simulink model "sm_backhoe"  (R2021b)
settings: Solver=ode23t  StartTime=0.0  StopTime=60  MaxStep=0.1  RelTol=1e-3  EnableMultiTasking=on
model workspace (MATLAB code in the model file):
  | cylinderGray = [0.6 0.6 0.6];
  | darkOrange = [0.8 0.5 0];
  | glassBlue = [0.2 0.2 1];
  | gray = [0.3 0.3 0.3];
  | orange = [0.8 0.65 0];
  | pistonGray = [0.4 0.4 0.4];
  | tireBlack = [0.1 0.1 0.1];
  | wheelGray = [0.6 0.6 0.6];
  | yellow = [0.8 0.8 0];
  | 
  | rhoGlass = 2500;
  | rhoRubber = 1500;
  | rhoSteel = 7800;
undefined symbols (not defined in the file): sigbuilder_block, X, Y, Z
libraries: sm_lib x161, sm_backhoe_lib x38, nesl_utility x9
(part 1 of 5)
Description:
  | Backhoe
  | 
  | This example shows a hydraulically actuated backhoe model with closed-loop PID control. The mechanism consists of a fixed vehicle model with a base mounting bracket. The bracket allows the backhoe arm to swivel left and right. Additionally, this arm has three rotational degrees of freedom for controlling the position of the bucket relative to the base swivel point.
  | 
  | The backhoe is actuated using pressure inputs to linear acting hydraulic cylinders. Pressure is controlled with decoupled PID controllers that  act on the error between measured and reference angular positions.
settings Model: Creator=The MathWorks, Inc.  LastModifiedBy=The MathWorks, Inc.
settings SolverCC: AlgebraicLoopSolver=TrustRegion  SolverResetMethod=Robust
settings DataIOCC: LimitDataPoints=on  SaveFormat=Array  SaveOutput=off  SaveTime=off  ReturnWorkspaceOutputs=off  Refine=3
settings OptimizationCC: ExpressionDepthLimit=2147483647  LifeSpan=inf
settings DebuggingCC: UnderspecifiedInitializationDetection=Classic  MergeDetectMultiDrivingBlocksExec=none  StateNameClashWarn=warning  SFUnexpectedBacktrackingDiag=warning  SFNoUnconditionalDefaultTransitionDiag=warning  SFExecutionAtInitializationDiag=none  SFMachineParentedDataDiag=warning  ArithmeticOperatorsInVariantConditions=warning
settings HardwareCC: ProdBitPerPointer=32  ProdBitPerSizeT=32  ProdBitPerPtrDiffT=32  ProdLargestAtomicFloat=None  ProdIntDivRoundTo=Undefined  ProdEndianess=Unspecified  ProdWordSize=32  ProdHWDeviceType=32-bit Generic
settings ModelReferenceCC: PropagateSignalLabelsOutOfModel=off
settings SFSimCC: SimUseLocalCustomCode=off  CustomCodeUndefinedFunction=UseInterfaceOnly
settings RTWCC: RTWUseLocalCustomCode=off
settings CodeAppCC: StateflowObjectComments=on
settings GRTTargetCC: TargetLangStandard=C89/C90 (ANSI)
settings ConfigComp: CovMetricSettings=dw  CovSaveCumulativeToWorkspaceVar=on  CovSaveSingleToWorkspaceVar=on  CovExternalEMLEnable=off  CovSFcnEnable=off
settings SimscapeCC: SimscapeNormalizeSystem=off  SimscapeLogType=all  SimscapeLogSimulationStatistics=on  SimscapeLogName=simlog_sm_backhoe  SimscapeLogLimitData=off
settings ConfigurationSet: Description=SimMechanics 2G
settings ExplorerConfigSet: InternalSimMechanicsExplorerSettings="<ExplorerConfiguration><canonicalview>default</canonicalview><TilePanel><TileInfo><Tiles Columns=\"1\" Count=\"1\" Rows=\"1\"><Column Left=\"2\" Weight=\"1\"/><Column Left=\"638\"/><Row Top=\"2\" Weight=\"1\"/><Row Top=\"570\"/><Tile Height=\"1\" Width=\"1\" X=\"0\" Y=\"0\"/></Tiles></TileInfo><SceneInfo><SceneViewer><BGColor><R>0.60000002384185791</R><G>0.60000002384185791</G><B>0.60000002384185791</B></BGColor><Camera><Position><X>17.081954992990738</X><Y>-26.191145003137979</Y><Z>19.643565568520032</Z></Position><Center><X>-1.4975646002791232</X><Y>-7.6116254098681191</Y><Z>1.0640459752315596</Z></Center><Up><X>-0.40824829046386307</X><Y>0.40824829046386307</Y><Z>0.81649658092772615</Z></Up><Left>-11.606539788284151</Left><Right>11.606539788284151</Right><Bottom>-11.304127508235643</Bottom><Top>11.304127508235643</Top></Camera></SceneViewer></SceneInfo></TilePanel></ExplorerConfiguration>"

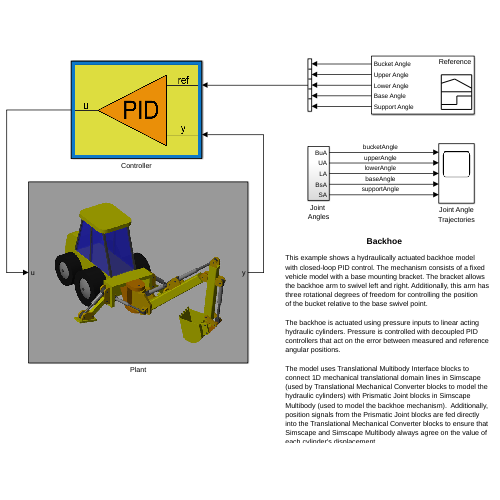
[thumbnail: Simulink's stored preview of the top-level diagram]
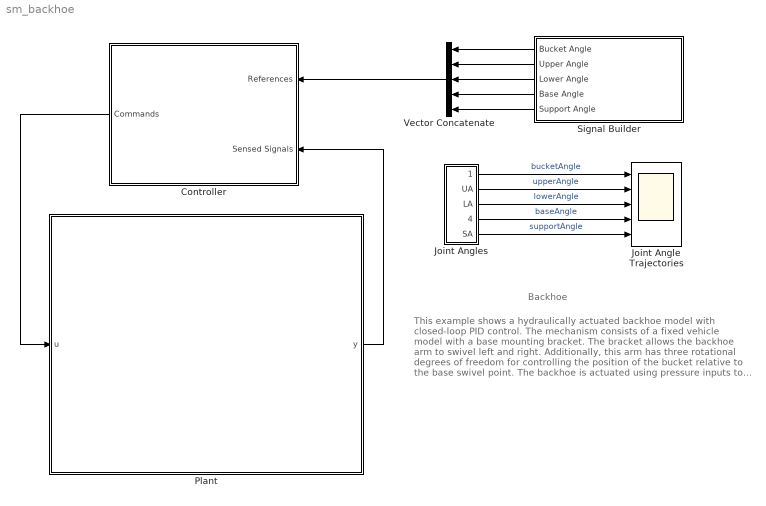
== system sm_backhoe ==
  note: Backhoe
  note: This example shows a hydraulically actuated backhoe model
      | with closed-loop PID control. The mechanism consists of a fixed
      | vehicle model with a base mounting bracket. The bracket allows
      | the backhoe arm to swivel left and right. Additionally, this arm has
      | three rotational degrees of freedom for controlling the position
      | of the bucket relative to the base swivel point.
      |
      | The backhoe is actuated using pressure inputs to linear acting
      | hydraulic cylinders. Pressure is controlled with decoupled PID
      | controllers that act on the error between measured and reference
      | angular positions.
      |
      | The model uses Translational Multibody Interface blocks to
      | connect 1D mechanical translational domain lines in Simscape (used by Translational Mechanical Converter blocks to model the hydraulic cylinders) with Prismatic Joint blocks in Simscape Multibody (used to model the backhoe mechanism).  Additionally, position signals from the Prismatic Joint blocks are fed directly into the Translational Mechanical Converter blocks to ensure that Simscape and Simscape Multibody always agree on the value of each cylinder's displacement.
  Controller : Subsystem
      mask Display: image(fullfile(matlabroot,'toolbox','physmod','sm','smdemos','backhoe','images','sm_backhoe_PIDmask.png'));
  Joint Angles : Subsystem
  Joint Angle Trajectories : Scope  NumInputPorts=5
  Plant : Subsystem
      mask Display:
      | image(fullfile(matlabroot,'toolbox','physmod','sm','smdemos','backhoe','images','sm_backhoe.png'));
      | port_label('input',1,'u');
      | port_label('output',1,'y');
  Signal Builder : Subsystem  Tag=STV Subsys  LoadFcn=sigbuilder_block('load');  StartFcn=sigbuilder_block('start');  StopFcn=sigbuilder_block('stop');  ClipboardFcn=sigbuilder_block('clipboard');  mask(Sigbuilder block){tuvar=[0:10]}
      mask help: Simulink:masks:SigbuilderBlock_MD
      mask init:
      | if ~strcmp(get_param(bdroot(gcbh),'SimulationStatus'),'stopped') tuvar = sigbuilder_block('maskInit'); end
      settings: CopyFcn=sigbuilder_block('copy');  DeleteFcn=sigbuilder_block('delete');  ModelCloseFcn=sigbuilder_block('modelClose');  PreSaveFcn=sigbuilder_block('preSave');  PauseFcn=sigbuilder_block('pause');  ContinueFcn=sigbuilder_block('continue');  NameChangeFcn=sigbuilder_block('namechange');  OpenFcn=sigbuilder_block('open',[252 212.25 471.75 399 ]);  CloseFcn=sigbuilder_block('close');
      mask Display: plot(0, 0, 100, 100,[2, 2, 32, 32, 2], [68, 8, 8, 68, 68],[32, 2], [38, 38], [32, 19, 2],[53, 60, 44], [32, 17, 17, 2],[16, 16, 31, 31]);txt = getActiveGroup(gcbh);text(2, 100, txt,'verticalAlignment', 'top');
  Vector Concatenate : Concatenate  NumInputs=5
  wires:
  Controller/1(Commands) -> Plant/1(u)
  Joint Angles/1(BuA) -> Joint Angle Trajectories/1  "bucketAngle"
  Joint Angles/2(UA) -> Joint Angle Trajectories/2  "upperAngle"
  Joint Angles/3(LA) -> Joint Angle Trajectories/3  "lowerAngle"
  Joint Angles/4(BsA) -> Joint Angle Trajectories/4  "baseAngle"
  Joint Angles/5(SA) -> Joint Angle Trajectories/5  "supportAngle"
  Plant/1(y) -> Controller/2(Sensed Signals)
  Vector Concatenate/1 -> Controller/1(References)
  Signal Builder/2(Upper Angle) -> Vector Concatenate/2
  Signal Builder/3(Lower Angle) -> Vector Concatenate/3
  Signal Builder/1(Bucket Angle) -> Vector Concatenate/1
  Signal Builder/5(Support Angle) -> Vector Concatenate/5
  Signal Builder/4(Base Angle) -> Vector Concatenate/4

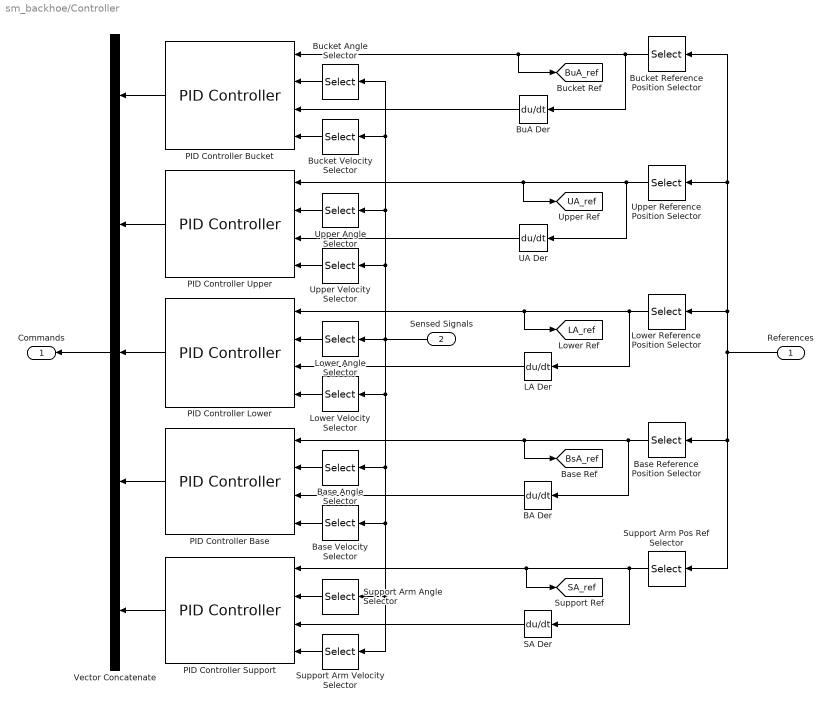
== system sm_backhoe/Controller ==
  References : Inport
  Sensed Signals : Inport  Port=2
  BA Der : Derivative
  Base Angle Selector : Selector  InputPortWidth=10  IndexOptions=Index vector (dialog)  Indices=7  OutputSizes=1
  Base Reference Position Selector : Selector  InputPortWidth=5  IndexOptions=Index vector (dialog)  Indices=4  OutputSizes=1
  Base Velocity Selector : Selector  InputPortWidth=10  IndexOptions=Index vector (dialog)  Indices=8  OutputSizes=1
  BuA Der : Derivative
  Bucket Angle Selector : Selector  InputPortWidth=10  IndexOptions=Index vector (dialog)  Indices=1  OutputSizes=1
  Bucket Reference Position Selector : Selector  InputPortWidth=5  IndexOptions=Index vector (dialog)  Indices=1  OutputSizes=1
  Bucket Velocity Selector : Selector  InputPortWidth=10  IndexOptions=Index vector (dialog)  Indices=2  OutputSizes=1
  LA Der : Derivative
  Lower Angle Selector : Selector  InputPortWidth=10  IndexOptions=Index vector (dialog)  Indices=5  OutputSizes=1
  Lower Reference Position Selector : Selector  InputPortWidth=5  IndexOptions=Index vector (dialog)  Indices=3  OutputSizes=1
  Lower Velocity Selector : Selector  InputPortWidth=10  IndexOptions=Index vector (dialog)  Indices=6  OutputSizes=1
  PID Controller Base : sm_backhoe_lib/PID Controller  upperLim=40  lowerLim=-40  Kp=65  Ki=10  Kd=10
      settings: SourceProductBaseCode=MS
  PID Controller Bucket : sm_backhoe_lib/PID Controller  upperLim=10  lowerLim=-120  Kp=50  Ki=2  Kd=3
      settings: SourceProductBaseCode=MS
  PID Controller Lower : sm_backhoe_lib/PID Controller  upperLim=40  lowerLim=-70  Kp=360  Ki=100  Kd=75
      settings: SourceProductBaseCode=MS
  PID Controller Support : sm_backhoe_lib/PID Controller  upperLim=-40  lowerLim=-100  Kp=40  Ki=1  Kd=2
      settings: SourceProductBaseCode=MS
  PID Controller Upper : sm_backhoe_lib/PID Controller  upperLim=60  lowerLim=-20  Kp=150  Ki=5  Kd=10
      settings: SourceProductBaseCode=MS
  SA Der : Derivative
  Support Arm Angle Selector : Selector  InputPortWidth=10  IndexOptions=Index vector (dialog)  Indices=9  OutputSizes=1
  Support Arm Velocity Selector : Selector  InputPortWidth=10  IndexOptions=Index vector (dialog)  Indices=10  OutputSizes=1
  Support Arm Pos Ref Selector : Selector  InputPortWidth=5  IndexOptions=Index vector (dialog)  Indices=5  OutputSizes=1
  UA Der : Derivative
  Upper Angle Selector : Selector  InputPortWidth=10  IndexOptions=Index vector (dialog)  Indices=3  OutputSizes=1
  Upper Reference Position Selector : Selector  InputPortWidth=5  IndexOptions=Index vector (dialog)  Indices=2  OutputSizes=1
  Upper Velocity Selector : Selector  InputPortWidth=10  IndexOptions=Index vector (dialog)  Indices=4  OutputSizes=1
  Vector Concatenate : Concatenate  NumInputs=5
  Commands : Outport
  tag scope: BsA_ref=global, BuA_ref=global, LA_ref=global, SA_ref=global, UA_ref=global
  wires:
  Vector Concatenate/1 -> Commands/1
  Sensed Signals/1 -> Support Arm Velocity Selector/1, Support Arm Angle Selector/1, Base Velocity Selector/1, Base Angle Selector/1, Lower Velocity Selector/1, Bucket Velocity Selector/1, Bucket Angle Selector/1, Upper Angle Selector/1, Upper Velocity Selector/1, Lower Angle Selector/1
  Upper Angle Selector/1 -> PID Controller Upper/2
  Base Angle Selector/1 -> PID Controller Base/2
  Support Arm Angle Selector/1 -> PID Controller Support/2
  Bucket Angle Selector/1 -> PID Controller Bucket/2
  Lower Angle Selector/1 -> PID Controller Lower/2
  References/1 -> Bucket Reference Position Selector/1, Upper Reference Position Selector/1, Lower Reference Position Selector/1, Support Arm Pos Ref Selector/1, Base Reference Position Selector/1
  PID Controller Support/1 -> Vector Concatenate/5
  Upper Reference Position Selector/1 -> UA Der/1, PID Controller Upper/1, [UA_ref]
  Lower Reference Position Selector/1 -> LA Der/1, [LA_ref], PID Controller Lower/1
  Base Reference Position Selector/1 -> BA Der/1, PID Controller Base/1, [BsA_ref]
  Support Arm Pos Ref Selector/1 -> SA Der/1, [SA_ref], PID Controller Support/1
  Bucket Reference Position Selector/1 -> BuA Der/1, [BuA_ref], PID Controller Bucket/1
  Support Arm Velocity Selector/1 -> PID Controller Support/4
  SA Der/1 -> PID Controller Support/3
  Base Velocity Selector/1 -> PID Controller Base/4
  BA Der/1 -> PID Controller Base/3
  PID Controller Base/1 -> Vector Concatenate/4
  Lower Velocity Selector/1 -> PID Controller Lower/4
  LA Der/1 -> PID Controller Lower/3
  Upper Velocity Selector/1 -> PID Controller Upper/4
  UA Der/1 -> PID Controller Upper/3
  Bucket Velocity Selector/1 -> PID Controller Bucket/4
  BuA Der/1 -> PID Controller Bucket/3
  PID Controller Lower/1 -> Vector Concatenate/3
  PID Controller Upper/1 -> Vector Concatenate/2
  PID Controller Bucket/1 -> Vector Concatenate/1

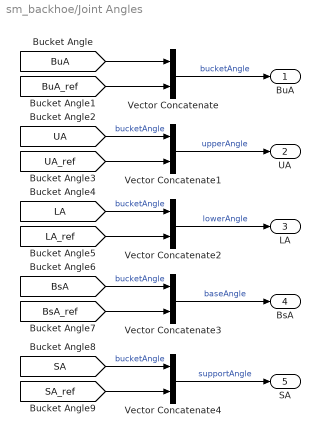
== system sm_backhoe/Joint Angles ==
  Vector Concatenate{,1..4} (5 alike) : Concatenate
  BuA : Outport
  UA : Outport  Port=2
  LA : Outport  Port=3
  BsA : Outport  Port=4
  SA : Outport  Port=5
  wires:
  Vector Concatenate1/1 -> UA/1  "upperAngle"
  Vector Concatenate2/1 -> LA/1  "lowerAngle"
  Vector Concatenate/1 -> BuA/1  "bucketAngle"
  Vector Concatenate3/1 -> BsA/1  "baseAngle"
  Vector Concatenate4/1 -> SA/1  "supportAngle"
  [BuA] -> Vector Concatenate/1
  [BuA_ref] -> Vector Concatenate/2
  [UA] -> Vector Concatenate1/1  "bucketAngle"
  [UA_ref] -> Vector Concatenate1/2
  [LA] -> Vector Concatenate2/1  "bucketAngle"
  [LA_ref] -> Vector Concatenate2/2
  [BsA] -> Vector Concatenate3/1  "bucketAngle"
  [BsA_ref] -> Vector Concatenate3/2
  [SA] -> Vector Concatenate4/1  "bucketAngle"
  [SA_ref] -> Vector Concatenate4/2

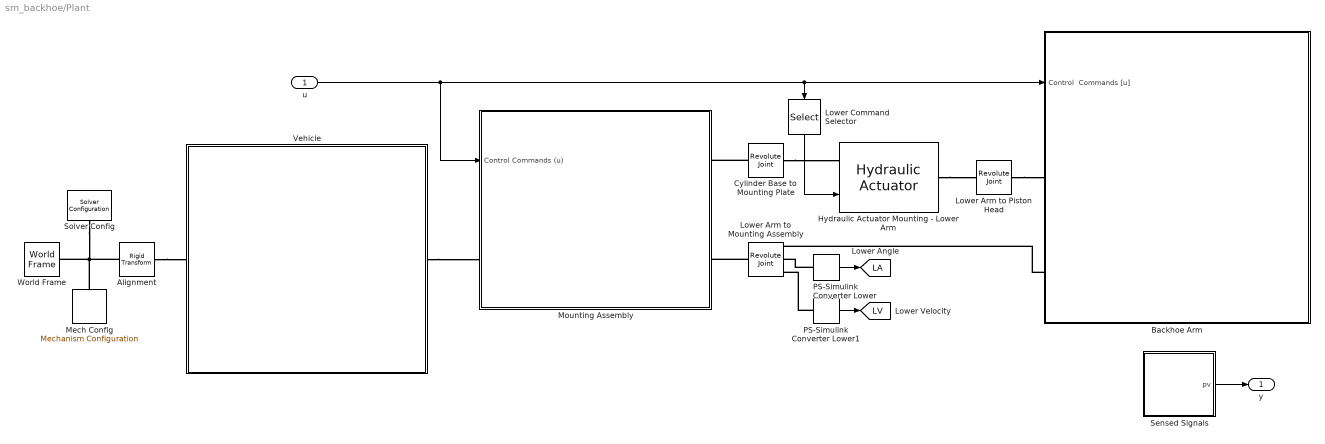
== system sm_backhoe/Plant ==
  u : Inport
  Alignment : sm_lib/Frames and Transforms/Rigid Transform  TranslationMethod=None  TranslationStandardOffset=0  TranslationLengthUnit=m  TranslationStandardAxis=+Z  TranslationCartesianOffset=[0 0 0]  TranslationROffset=0  TranslationROffsetUnits=m  TranslationZOffset=0  TranslationZOffsetUnits=m  TranslationThetaOffset=0  TranslationThetaOffsetUnits=deg  RotationMethod=AlignedAxes  RotationAngleUnits=deg  RotationStandardAxis=+X  RotationAngle=90  RotationArbitraryAxis=[0 0 1]  FollAlignAxisA=+X  BaseAlignAxisA=+X  FollAlignAxisB=+Y  BaseAlignAxisB=+Z  RotationSequenceAxes=FollowerAxes  RotationSequence=XYX  RotationSequenceAngles=[0 0 0]  RotationSequenceAnglesUnits=deg  RotationMatrix=[1 0 0; 0 1 0; 0 0 1]
  Backhoe Arm : Subsystem
      mask Display:
      | image(fullfile(matlabroot,'toolbox','physmod','sm','smdemos','backhoe','images','sm_backhoe_arms.png'));
      | port_label('lconn',2,'MA');
      | port_label('lconn',1,'LC');
      | port_label('input',1,'u');
  Cylinder Base to Mounting Plate : sm_lib/Joints/Revolute Joint  JointMode=Normal  SenseConstraintForce=off  SenseConstraintForceX=off  SenseConstraintForceY=off  SenseConstraintForceZ=off  SenseConstraintTorque=off  SenseConstraintTorqueX=off  SenseConstraintTorqueY=off  SenseConstraintTorqueZ=off  SenseTotalForce=off  SenseTotalForceX=off  SenseTotalForceY=off  SenseTotalForceZ=off  SenseTotalTorque=off  SenseTotalTorqueX=off  SenseTotalTorqueY=off  SenseTotalTorqueZ=off  CompositeWrenchDir=FollowerOnBase  CompositeWrenchFrame=BaseFrame  EquilibriumPosition=0  EquilibriumPositionUnits=deg  SpringStiffness=0  SpringStiffnessUnits=N*m/deg  DampingCoefficient=0  DampingCoefficientUnits=N*m/(deg/s)  TorqueActuationMode=NoTorque  MotionActuationMode=ComputedMotion  SensePosition=off  SenseVelocity=off  SenseAcceleration=off  SenseTorqueForce=off  SenseLowerLimitTorqueForce=off  SenseUpperLimitTorqueForce=off  LowerLimitSpecify=off  LowerLimitBound=-90  LowerLimitBoundUnits=deg  LowerLimitStiffness=1e4  LowerLimitStiffnessUnits=N*m/deg  LowerLimitDamping=10  LowerLimitDampingUnits=N*m/(deg/s)  LowerLimitTransitionRegionWidth=0.1  LowerLimitTransitionRegionWidthUnits=deg  UpperLimitSpecify=off  UpperLimitBound=90  UpperLimitBoundUnits=deg  UpperLimitStiffness=1e4  UpperLimitStiffnessUnits=N*m/deg  UpperLimitDamping=10  UpperLimitDampingUnits=N*m/(deg/s)  UpperLimitTransitionRegionWidth=0.1  UpperLimitTransitionRegionWidthUnits=deg  PositionTargetSpecify=off  PositionTargetPriority=Low  PositionTargetValue=-45  PositionTargetValueUnits=deg  VelocityTargetSpecify=off  VelocityTargetPriority=High  VelocityTargetValue=0  VelocityTargetValueUnits=deg/s
  Hydraulic Actuator Mounting - Lower Arm : sm_backhoe_lib/Hydraulic Actuator  Lcyl=1.85  Rcyl=0.2  Lbase=0.65  Wbase=0.425  Rbp=0.075  Lbp=0.8  circlePointsCyl=25  circlePointsCylB=25  Lpist=1.85  Rpist=0.12  Whead=0.35  Lhead=0.65  Rhp=0.075  Lhp=0.9  circlePointsPist=25  cylColor=cylinderGray  rhoCyl=rhoSteel  pistColor=pistonGray  rhoPist=rhoSteel  connColor=gray  rhoConn=rhoSteel
      settings: SourceProductBaseCode=MS
  Lower Arm to Mounting Assembly : sm_lib/Joints/Revolute Joint  JointMode=Normal  SenseConstraintForce=off  SenseConstraintForceX=off  SenseConstraintForceY=off  SenseConstraintForceZ=off  SenseConstraintTorque=off  SenseConstraintTorqueX=off  SenseConstraintTorqueY=off  SenseConstraintTorqueZ=off  SenseTotalForce=off  SenseTotalForceX=off  SenseTotalForceY=off  SenseTotalForceZ=off  SenseTotalTorque=off  SenseTotalTorqueX=off  SenseTotalTorqueY=off  SenseTotalTorqueZ=off  CompositeWrenchDir=FollowerOnBase  CompositeWrenchFrame=BaseFrame  EquilibriumPosition=0  EquilibriumPositionUnits=deg  SpringStiffness=0  SpringStiffnessUnits=N*m/deg  DampingCoefficient=0  DampingCoefficientUnits=N*m/(deg/s)  TorqueActuationMode=NoTorque  MotionActuationMode=ComputedMotion  SensePosition=on  SenseVelocity=on  SenseAcceleration=off  SenseTorqueForce=off  SenseLowerLimitTorqueForce=off  SenseUpperLimitTorqueForce=off  LowerLimitSpecify=off  LowerLimitBound=-90  LowerLimitBoundUnits=deg  LowerLimitStiffness=1e4  LowerLimitStiffnessUnits=N*m/deg  LowerLimitDamping=10  LowerLimitDampingUnits=N*m/(deg/s)  LowerLimitTransitionRegionWidth=0.1  LowerLimitTransitionRegionWidthUnits=deg  UpperLimitSpecify=off  UpperLimitBound=90  UpperLimitBoundUnits=deg  UpperLimitStiffness=1e4  UpperLimitStiffnessUnits=N*m/deg  UpperLimitDamping=10  UpperLimitDampingUnits=N*m/(deg/s)  UpperLimitTransitionRegionWidth=0.1  UpperLimitTransitionRegionWidthUnits=deg  PositionTargetSpecify=on  PositionTargetPriority=High  PositionTargetValue=-60  PositionTargetValueUnits=deg  VelocityTargetSpecify=off  VelocityTargetPriority=High  VelocityTargetValue=0  VelocityTargetValueUnits=deg/s
  Lower Arm to Piston Head : sm_lib/Joints/Revolute Joint  JointMode=Normal  SenseConstraintForce=off  SenseConstraintForceX=off  SenseConstraintForceY=off  SenseConstraintForceZ=off  SenseConstraintTorque=off  SenseConstraintTorqueX=off  SenseConstraintTorqueY=off  SenseConstraintTorqueZ=off  SenseTotalForce=off  SenseTotalForceX=off  SenseTotalForceY=off  SenseTotalForceZ=off  SenseTotalTorque=off  SenseTotalTorqueX=off  SenseTotalTorqueY=off  SenseTotalTorqueZ=off  CompositeWrenchDir=FollowerOnBase  CompositeWrenchFrame=BaseFrame  EquilibriumPosition=0  EquilibriumPositionUnits=deg  SpringStiffness=0  SpringStiffnessUnits=N*m/deg  DampingCoefficient=0  DampingCoefficientUnits=N*m/(deg/s)  TorqueActuationMode=NoTorque  MotionActuationMode=ComputedMotion  SensePosition=off  SenseVelocity=off  SenseAcceleration=off  SenseTorqueForce=off  SenseLowerLimitTorqueForce=off  SenseUpperLimitTorqueForce=off  LowerLimitSpecify=off  LowerLimitBound=-90  LowerLimitBoundUnits=deg  LowerLimitStiffness=1e4  LowerLimitStiffnessUnits=N*m/deg  LowerLimitDamping=10  LowerLimitDampingUnits=N*m/(deg/s)  LowerLimitTransitionRegionWidth=0.1  LowerLimitTransitionRegionWidthUnits=deg  UpperLimitSpecify=off  UpperLimitBound=90  UpperLimitBoundUnits=deg  UpperLimitStiffness=1e4  UpperLimitStiffnessUnits=N*m/deg  UpperLimitDamping=10  UpperLimitDampingUnits=N*m/(deg/s)  UpperLimitTransitionRegionWidth=0.1  UpperLimitTransitionRegionWidthUnits=deg  PositionTargetSpecify=off  PositionTargetPriority=Low  PositionTargetValue=-45  PositionTargetValueUnits=deg  VelocityTargetSpecify=off  VelocityTargetPriority=High  VelocityTargetValue=0  VelocityTargetValueUnits=deg/s
  Lower Command Selector : Selector  InputPortWidth=5  IndexOptions=Index vector (dialog)  Indices=3  OutputSizes=1
  Mech Config : sm_lib/Utilities/Mechanism Configuration  UniformGravity=Constant  GravityVector=[0 0 -9.81]  GravityUnits=m/s^2  LinearizationDelta=0.001  JointModeTransitionNonlinearIterations=2
  Mounting Assembly : Subsystem
      mask Display:
      | image(fullfile(matlabroot,'toolbox','physmod','sm','smdemos','backhoe','images','sm_backhoe_mountingassembly.png'))
      | port_label('input',1,'u')
      | port_label('lconn',1,'V')
      | port_label('rconn',1,'LH')
      | port_label('rconn',2,'LA')
  PS-Simulink Converter Lower : nesl_utility/PS-Simulink Converter  PhysicalDomain=network_engine_domain  SubClassName=ps_output  LeftPortType=input  RightPortType=output  PseudoPeriodic=off  Frequencies=[]  Unit=deg  AffineConversion=off
      settings: SourceProductBaseCode=PW,SS
  PS-Simulink Converter Lower1 : nesl_utility/PS-Simulink Converter  PhysicalDomain=network_engine_domain  SubClassName=ps_output  LeftPortType=input  RightPortType=output  PseudoPeriodic=off  Frequencies=[]  Unit=deg/s  AffineConversion=off
      settings: SourceProductBaseCode=PW,SS
  Sensed Signals : Subsystem
  Solver Config : nesl_utility/Solver Configuration  PhysicalDomain=network_engine_domain  SubClassName=solver  LeftPortType=input  RightPortType=generic  Tones=[]  Harmonics=[]  SimulateNoise=off  Profile=off  UseLocalSampling=off  EnableSwitchedLinearOptims=on  FrequencyDomain=off  UseCCode=off  RelTol=0.001  AbsTol=1e-06  MinStep=1e-09  ToWorkspace=off  RevertToSquareIcSolve=off  NumHomotopyIterations=100  PhasorMode=off  PhasorModeNumHarmonics=1  DoDC=off  ResidualTolerance=1e-9  UseLocalSolver=off  LocalSolverChoice=NE_BACKWARD_EULER_ADVANCER  LocalSolverSampleTime=1e-3  DoFixedCost=off  MaxNonlinIter=3  MaxModeIter=2  ComputeImpulses=off  ImpulseIterations=2  LinearAlgebra=Sparse  EquationFormulation=NE_TIME_EF  DelaysMemoryBudget=1024  AutomaticFiltering=on  FilteringTimeConstant=0.001  PartitionStorageMethod=AS_NEEDED  PartitionMemoryBudget=1024  PartitionMethod=FAST
      settings: SourceProductBaseCode=PW,SS
  Vehicle : Subsystem
      mask Display:
      | image(fullfile(matlabroot,'toolbox','physmod','sm','smdemos','backhoe','images','sm_backhoe_vehicle.png'));
      | port_label('lconn',1,'MA');
      | port_label('rconn',1,'G');
  World Frame : sm_lib/Frames and Transforms/World Frame
  y : Outport
  tag scope: LA=global, LV=global
  wires:
  u/1 -> Lower Command Selector/1, Backhoe Arm/1(Control  Commands [u]), Mounting Assembly/1(Control Commands (u))
  PS-Simulink Converter Lower/1 -> [LA]
  Lower Command Selector/1 -> Hydraulic Actuator Mounting - Lower Arm/1
  PS-Simulink Converter Lower1/1 -> [LV]
  Sensed Signals/1(pv) -> y/1
  connections:
  Alignment/LConn1 -- World Frame/RConn1 -- Solver Config/RConn1 -- Mech Config/RConn1
  Alignment/RConn1 -- Vehicle/RConn1
  PS-Simulink Converter Lower/LConn1 -- Lower Arm to Mounting Assembly/RConn2
  Vehicle/LConn1 -- Mounting Assembly/LConn1
  Cylinder Base to Mounting Plate/LConn1 -- Mounting Assembly/RConn1
  Lower Arm to Mounting Assembly/LConn1 -- Mounting Assembly/RConn2
  Backhoe Arm/LConn2 -- Lower Arm to Mounting Assembly/RConn1
  Cylinder Base to Mounting Plate/RConn1 -- Hydraulic Actuator Mounting - Lower Arm/LConn1
  Hydraulic Actuator Mounting - Lower Arm/RConn1 -- Lower Arm to Piston Head/LConn1
  Lower Arm to Piston Head/RConn1 -- Backhoe Arm/LConn1
  PS-Simulink Converter Lower1/LConn1 -- Lower Arm to Mounting Assembly/RConn3

== system sm_backhoe/Signal Builder ==
  Demux : Demux  Tag=STV Demux  Outputs=5
      settings: DisplayOption=none
  FromWs : FromWorkspace  Tag=STV FromWs  VariableName=tuvar  OutputAfterFinalValue=Holding final value
      SigBuilderData=|
      | common.afterFinalStr = 'Hold final value'
      | common.sampleTime = '0'
      | dataSet.timeRange = [0 60]
      | dataSet.name = 'Reference'
      | sbobj.Groups.Name = 'Reference'
      | sbobj.Groups.Signals(1).Name = 'Bucket Angle'
      | sbobj.Groups.Signals(1).XData = [0 7 11 24 28.5 40 42 48 51 60]
      | sbobj.Groups.Signals(1).YData = [0 0 -90 -90 0 0 -105 -105 0 0]
      | sbobj.Groups.Signals(2).Name = 'Upper Angle'
      | sbobj.Groups.Signals(2).XData = [0 12.5 25 30 34 38 40 42 48 52 60]
      | sbobj.Groups.Signals(2).YData = [50 50 -20 -20 17 55 55 20 20 55 55]
      | sbobj.Groups.Signals(3).Name = 'Lower Angle'
      | sbobj.Groups.Signals(3).XData = [0 15 27.5 30 36 40 60]
      | sbobj.Groups.Signals(3).YData = [-60 -60 -15 -15 -60 -60 -60]
      | sbobj.Groups.Signals(4).Name = 'Base Angle'
      | sbobj.Groups.Signals(4).XData = [0 6 10 32.5 40 48 53 60]
      | sbobj.Groups.Signals(4).YData = [0 -0.01 -30 -30 30 30 0.01 0]
      | sbobj.Groups.Signals(5).Name = 'Support Angle'
      | sbobj.Groups.Signals(5).XData = [0 1 5 55 59 60]
      | sbobj.Groups.Signals(5).YData = [-90 -90 -45 -45 -90 -90]
      | sbobj.Groups.TimeRange = [0 60]
  Bucket Angle : Outport  Tag=STV Outport
  Upper Angle : Outport  Tag=STV Outport  Port=2
  Lower Angle : Outport  Tag=STV Outport  Port=3
  Base Angle : Outport  Tag=STV Outport  Port=4
  Support Angle : Outport  Tag=STV Outport  Port=5
  wires:
  Demux/1 -> Bucket Angle/1
  FromWs/1 -> Demux/1
  Demux/2 -> Upper Angle/1
  Demux/3 -> Lower Angle/1
  Demux/4 -> Base Angle/1
  Demux/5 -> Support Angle/1

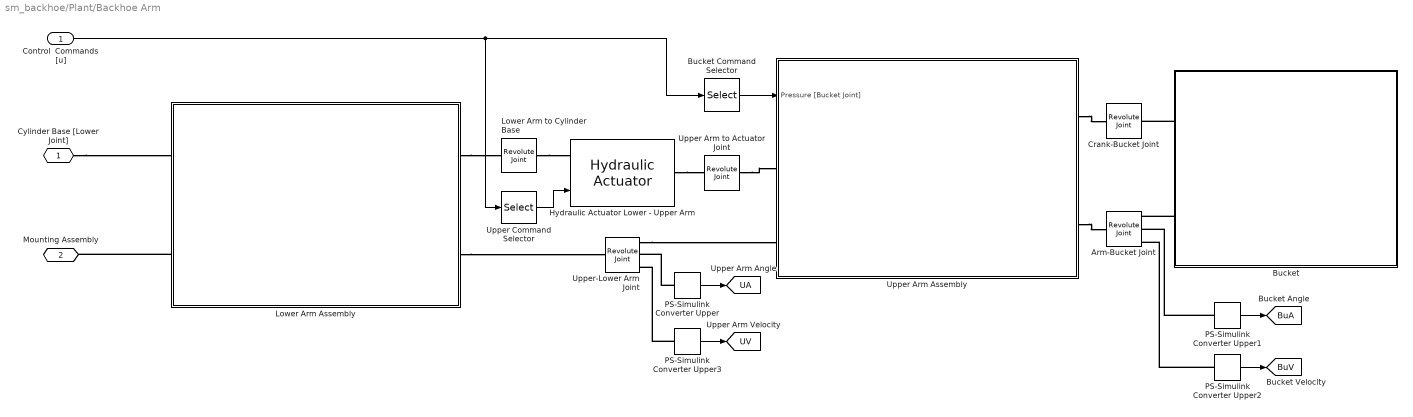
== system sm_backhoe/Plant/Backhoe Arm ==
  Control  Commands [u] : Inport
  Arm-Bucket Joint : sm_lib/Joints/Revolute Joint  JointMode=Normal  SenseConstraintForce=off  SenseConstraintForceX=off  SenseConstraintForceY=off  SenseConstraintForceZ=off  SenseConstraintTorque=off  SenseConstraintTorqueX=off  SenseConstraintTorqueY=off  SenseConstraintTorqueZ=off  SenseTotalForce=off  SenseTotalForceX=off  SenseTotalForceY=off  SenseTotalForceZ=off  SenseTotalTorque=off  SenseTotalTorqueX=off  SenseTotalTorqueY=off  SenseTotalTorqueZ=off  CompositeWrenchDir=FollowerOnBase  CompositeWrenchFrame=BaseFrame  EquilibriumPosition=0  EquilibriumPositionUnits=deg  SpringStiffness=0  SpringStiffnessUnits=N*m/deg  DampingCoefficient=0  DampingCoefficientUnits=N*m/(deg/s)  TorqueActuationMode=NoTorque  MotionActuationMode=ComputedMotion  SensePosition=on  SenseVelocity=on  SenseAcceleration=off  SenseTorqueForce=off  SenseLowerLimitTorqueForce=off  SenseUpperLimitTorqueForce=off  LowerLimitSpecify=off  LowerLimitBound=-90  LowerLimitBoundUnits=deg  LowerLimitStiffness=1e4  LowerLimitStiffnessUnits=N*m/deg  LowerLimitDamping=10  LowerLimitDampingUnits=N*m/(deg/s)  LowerLimitTransitionRegionWidth=0.1  LowerLimitTransitionRegionWidthUnits=deg  UpperLimitSpecify=off  UpperLimitBound=90  UpperLimitBoundUnits=deg  UpperLimitStiffness=1e4  UpperLimitStiffnessUnits=N*m/deg  UpperLimitDamping=10  UpperLimitDampingUnits=N*m/(deg/s)  UpperLimitTransitionRegionWidth=0.1  UpperLimitTransitionRegionWidthUnits=deg  PositionTargetSpecify=on  PositionTargetPriority=High  PositionTargetValue=0  PositionTargetValueUnits=deg  VelocityTargetSpecify=off  VelocityTargetPriority=High  VelocityTargetValue=0  VelocityTargetValueUnits=deg/s
  Bucket : Subsystem  mask(Bucket){plateSide=1.2, plateFilletR=0.2, plateDist=1.2, plateWidth=0.2, plateHoleR=0.075, bucketHeight=2, bucketLength=2, bucketThickness=0.05, bucketUpper=1.3, bucketLower=2, chordAngle=pi/6, toothLength=0.25, toothWidth=0.2, toothTip=0.025, circlePoints=45, bucketColor=yellow, bracketColor=yellow, rho=rhoSteel}
      mask prompts: plateSide "Wplate (m)"; plateFilletR "Rfillet (m)"; plateDist "Dplate (m)"; plateWidth "Tplate (m)"; plateHoleR "Rpin (m)"; bucketHeight "Hbucket (m)"; bucketLength "Wbucket (m)"; bucketThickness "Tbucket (m)"; bucketUpper "Wupper (m)"; bucketLower "Wlower (m)"; chordAngle "alpha (radians)"; toothLength "Ltooth (m)"; toothWidth "Wtooth (m)"; toothTip "Ttooth (m)"; circlePoints "Circle Resolution  (pts/rev)"; bucketColor "Bucket Color"; bracketColor "Bracket Color"; rho "Density (kg/m^3)"
      mask help:
      | Consists of the backhoe bucket assembly with attachment frame.
      |
      | Attachment points are:
      | CA: Center point of the Crank Arm link pin.
      | UA: Center Point of the Upper Arm link pin.
      | Both points are configured for Revolute joints.
      |
      | Click on Help to view a schematic of the bucket, its configurable dimension parameters and attachment points (in red).
      mask init:
      | bucketRadius = bucketHeight/(2*cos(chordAngle));
      | 
      | % Bucket Back
      | bucketBack = [];
      | % Outer wall
      | for i = 0:circlePoints;
      |    angle = (-pi/2+chordAngle) + (pi - 2*chordAngle)*(i/circlePoints);
      |    bucketBack = [bucketBack; ...
      |        (bucketRadius*cos(angle)-bucketRadius*sin(chordAngle)) ...
      |         bucketRadius*sin(angle)];
      | end
      | 
      | % Inner Wall
      | beta = acos( ( (bucketRadius*cos(chordAngle) - bucketThickness/cos(chordAngle)) ...
      |                    /(bucketRadius-bucketThickness)) );
      | for i = 0:circlePoints;
      |    angle = (pi/2 - beta) - (pi-2*beta)*(i/circlePoints);
      |    bucketBack = [bucketBack; ...
      |        ((bucketRadius-bucketThickness)*cos(angle)-bucketRadius*sin(chordAngle)) ... 
      |        (bucketRadius-bucketThickness)*sin(angle)];
      | end
      | 
      | bucketBack = [bucketBack; ...
      |               -bucketLower -(bucketHeight/2-bucketThickness);...
      |               -bucketLower -bucketHeight/2];
      |           
      | % Uncomment below to plot the cross-sections. 
      | % close all
      | % figure
      | % plot(bucketBack(:,1),bucketBack(:,2));
      mask Help: web(fullfile(matlabroot,'toolbox','physmod','sm','smdemos','backhoe','demohelp','sm_backhoe_bucket.html'));
      mask Display:
      | image(fullfile(matlabroot,'toolbox','physmod','sm','smdemos','backhoe','images','sm_backhoe_bucket.png'));
      | port_label('rconn',1,'CA');
      | port_label('rconn',2,'UA');
  Bucket Command Selector : Selector  InputPortWidth=5  IndexOptions=Index vector (dialog)  Indices=1  OutputSizes=1
  Crank-Bucket Joint : sm_lib/Joints/Revolute Joint  JointMode=Normal  SenseConstraintForce=off  SenseConstraintForceX=off  SenseConstraintForceY=off  SenseConstraintForceZ=off  SenseConstraintTorque=off  SenseConstraintTorqueX=off  SenseConstraintTorqueY=off  SenseConstraintTorqueZ=off  SenseTotalForce=off  SenseTotalForceX=off  SenseTotalForceY=off  SenseTotalForceZ=off  SenseTotalTorque=off  SenseTotalTorqueX=off  SenseTotalTorqueY=off  SenseTotalTorqueZ=off  CompositeWrenchDir=FollowerOnBase  CompositeWrenchFrame=BaseFrame  EquilibriumPosition=0  EquilibriumPositionUnits=deg  SpringStiffness=0  SpringStiffnessUnits=N*m/deg  DampingCoefficient=0  DampingCoefficientUnits=N*m/(deg/s)  TorqueActuationMode=NoTorque  MotionActuationMode=ComputedMotion  SensePosition=off  SenseVelocity=off  SenseAcceleration=off  SenseTorqueForce=off  SenseLowerLimitTorqueForce=off  SenseUpperLimitTorqueForce=off  LowerLimitSpecify=off  LowerLimitBound=-90  LowerLimitBoundUnits=deg  LowerLimitStiffness=1e4  LowerLimitStiffnessUnits=N*m/deg  LowerLimitDamping=10  LowerLimitDampingUnits=N*m/(deg/s)  LowerLimitTransitionRegionWidth=0.1  LowerLimitTransitionRegionWidthUnits=deg  UpperLimitSpecify=off  UpperLimitBound=90  UpperLimitBoundUnits=deg  UpperLimitStiffness=1e4  UpperLimitStiffnessUnits=N*m/deg  UpperLimitDamping=10  UpperLimitDampingUnits=N*m/(deg/s)  UpperLimitTransitionRegionWidth=0.1  UpperLimitTransitionRegionWidthUnits=deg  PositionTargetSpecify=off  PositionTargetPriority=Low  PositionTargetValue=0  PositionTargetValueUnits=deg  VelocityTargetSpecify=off  VelocityTargetPriority=High  VelocityTargetValue=0  VelocityTargetValueUnits=deg/s
  Hydraulic Actuator Lower - Upper Arm : sm_backhoe_lib/Hydraulic Actuator  Lcyl=2.25  Rcyl=0.2  Lbase=0.65  Wbase=0.425  Rbp=0.075  Lbp=0.8  circlePointsCyl=25  circlePointsCylB=25  Lpist=2.25  Rpist=0.12  Whead=0.35  Lhead=0.65  Rhp=0.075  Lhp=0.9  circlePointsPist=25  cylColor=cylinderGray  rhoCyl=rhoSteel  pistColor=pistonGray  rhoPist=rhoSteel  connColor=gray  rhoConn=rhoSteel
      settings: SourceProductBaseCode=MS
  Lower Arm Assembly : Subsystem
      mask Display:
      | image(fullfile(matlabroot,'toolbox','physmod','sm','smdemos','backhoe','images','sm_backhoe_lowerassembly.png'));
      | port_label('lconn',1,'LH');
      | port_label('lconn',2,'MA');
      | port_label('rconn',1,'UC');
      | port_label('rconn',2,'UA');
  Lower Arm to Cylinder Base : sm_lib/Joints/Revolute Joint  JointMode=Normal  SenseConstraintForce=off  SenseConstraintForceX=off  SenseConstraintForceY=off  SenseConstraintForceZ=off  SenseConstraintTorque=off  SenseConstraintTorqueX=off  SenseConstraintTorqueY=off  SenseConstraintTorqueZ=off  SenseTotalForce=off  SenseTotalForceX=off  SenseTotalForceY=off  SenseTotalForceZ=off  SenseTotalTorque=off  SenseTotalTorqueX=off  SenseTotalTorqueY=off  SenseTotalTorqueZ=off  CompositeWrenchDir=FollowerOnBase  CompositeWrenchFrame=BaseFrame  EquilibriumPosition=0  EquilibriumPositionUnits=deg  SpringStiffness=0  SpringStiffnessUnits=N*m/deg  DampingCoefficient=0  DampingCoefficientUnits=N*m/(deg/s)  TorqueActuationMode=NoTorque  MotionActuationMode=ComputedMotion  SensePosition=off  SenseVelocity=off  SenseAcceleration=off  SenseTorqueForce=off  SenseLowerLimitTorqueForce=off  SenseUpperLimitTorqueForce=off  LowerLimitSpecify=off  LowerLimitBound=-90  LowerLimitBoundUnits=deg  LowerLimitStiffness=1e4  LowerLimitStiffnessUnits=N*m/deg  LowerLimitDamping=10  LowerLimitDampingUnits=N*m/(deg/s)  LowerLimitTransitionRegionWidth=0.1  LowerLimitTransitionRegionWidthUnits=deg  UpperLimitSpecify=off  UpperLimitBound=90  UpperLimitBoundUnits=deg  UpperLimitStiffness=1e4  UpperLimitStiffnessUnits=N*m/deg  UpperLimitDamping=10  UpperLimitDampingUnits=N*m/(deg/s)  UpperLimitTransitionRegionWidth=0.1  UpperLimitTransitionRegionWidthUnits=deg  PositionTargetSpecify=on  PositionTargetPriority=Low  PositionTargetValue=90  PositionTargetValueUnits=deg  VelocityTargetSpecify=off  VelocityTargetPriority=High  VelocityTargetValue=0  VelocityTargetValueUnits=deg/s
  PS-Simulink Converter Upper : nesl_utility/PS-Simulink Converter  PhysicalDomain=network_engine_domain  SubClassName=ps_output  LeftPortType=input  RightPortType=output  PseudoPeriodic=off  Frequencies=[]  Unit=deg  AffineConversion=off
      settings: SourceProductBaseCode=PW,SS
  PS-Simulink Converter Upper1 : nesl_utility/PS-Simulink Converter  PhysicalDomain=network_engine_domain  SubClassName=ps_output  LeftPortType=input  RightPortType=output  PseudoPeriodic=off  Frequencies=[]  Unit=deg  AffineConversion=off
      settings: SourceProductBaseCode=PW,SS
  PS-Simulink Converter Upper2 : nesl_utility/PS-Simulink Converter  PhysicalDomain=network_engine_domain  SubClassName=ps_output  LeftPortType=input  RightPortType=output  PseudoPeriodic=off  Frequencies=[]  Unit=deg/s  AffineConversion=off
      settings: SourceProductBaseCode=PW,SS
  PS-Simulink Converter Upper3 : nesl_utility/PS-Simulink Converter  PhysicalDomain=network_engine_domain  SubClassName=ps_output  LeftPortType=input  RightPortType=output  PseudoPeriodic=off  Frequencies=[]  Unit=deg/s  AffineConversion=off
      settings: SourceProductBaseCode=PW,SS
  Upper Arm Assembly : Subsystem
      mask Display:
      | image(fullfile(matlabroot,'toolbox','physmod','sm','smdemos','backhoe','images','sm_backhoe_upperassembly_actuator.png'));
      | port_label('input',1,'PB');
      | port_label('lconn',2,'LA');
      | port_label('lconn',1,'UH');
      | port_label('rconn',1,'BC');
      | port_label('rconn',2,'B');
  Upper Arm to Actuator Joint : sm_lib/Joints/Revolute Joint  JointMode=Normal  SenseConstraintForce=off  SenseConstraintForceX=off  SenseConstraintForceY=off  SenseConstraintForceZ=off  SenseConstraintTorque=off  SenseConstraintTorqueX=off  SenseConstraintTorqueY=off  SenseConstraintTorqueZ=off  SenseTotalForce=off  SenseTotalForceX=off  SenseTotalForceY=off  SenseTotalForceZ=off  SenseTotalTorque=off  SenseTotalTorqueX=off  SenseTotalTorqueY=off  SenseTotalTorqueZ=off  CompositeWrenchDir=FollowerOnBase  CompositeWrenchFrame=BaseFrame  EquilibriumPosition=0  EquilibriumPositionUnits=deg  SpringStiffness=0  SpringStiffnessUnits=N*m/deg  DampingCoefficient=0  DampingCoefficientUnits=N*m/(deg/s)  TorqueActuationMode=NoTorque  MotionActuationMode=ComputedMotion  SensePosition=off  SenseVelocity=off  SenseAcceleration=off  SenseTorqueForce=off  SenseLowerLimitTorqueForce=off  SenseUpperLimitTorqueForce=off  LowerLimitSpecify=off  LowerLimitBound=-90  LowerLimitBoundUnits=deg  LowerLimitStiffness=1e4  LowerLimitStiffnessUnits=N*m/deg  LowerLimitDamping=10  LowerLimitDampingUnits=N*m/(deg/s)  LowerLimitTransitionRegionWidth=0.1  LowerLimitTransitionRegionWidthUnits=deg  UpperLimitSpecify=off  UpperLimitBound=90  UpperLimitBoundUnits=deg  UpperLimitStiffness=1e4  UpperLimitStiffnessUnits=N*m/deg  UpperLimitDamping=10  UpperLimitDampingUnits=N*m/(deg/s)  UpperLimitTransitionRegionWidth=0.1  UpperLimitTransitionRegionWidthUnits=deg  PositionTargetSpecify=off  PositionTargetPriority=High  PositionTargetValue=0  PositionTargetValueUnits=deg  VelocityTargetSpecify=off  VelocityTargetPriority=High  VelocityTargetValue=0  VelocityTargetValueUnits=deg/s
  Upper Command Selector : Selector  InputPortWidth=5  IndexOptions=Index vector (dialog)  Indices=2  OutputSizes=1
  Upper-Lower Arm Joint : sm_lib/Joints/Revolute Joint  JointMode=Normal  SenseConstraintForce=off  SenseConstraintForceX=off  SenseConstraintForceY=off  SenseConstraintForceZ=off  SenseConstraintTorque=off  SenseConstraintTorqueX=off  SenseConstraintTorqueY=off  SenseConstraintTorqueZ=off  SenseTotalForce=off  SenseTotalForceX=off  SenseTotalForceY=off  SenseTotalForceZ=off  SenseTotalTorque=off  SenseTotalTorqueX=off  SenseTotalTorqueY=off  SenseTotalTorqueZ=off  CompositeWrenchDir=FollowerOnBase  CompositeWrenchFrame=BaseFrame  EquilibriumPosition=0  EquilibriumPositionUnits=deg  SpringStiffness=0  SpringStiffnessUnits=N*m/deg  DampingCoefficient=0  DampingCoefficientUnits=N*m/(deg/s)  TorqueActuationMode=NoTorque  MotionActuationMode=ComputedMotion  SensePosition=on  SenseVelocity=on  SenseAcceleration=off  SenseTorqueForce=off  SenseLowerLimitTorqueForce=off  SenseUpperLimitTorqueForce=off  LowerLimitSpecify=off  LowerLimitBound=-90  LowerLimitBoundUnits=deg  LowerLimitStiffness=1e4  LowerLimitStiffnessUnits=N*m/deg  LowerLimitDamping=10  LowerLimitDampingUnits=N*m/(deg/s)  LowerLimitTransitionRegionWidth=0.1  LowerLimitTransitionRegionWidthUnits=deg  UpperLimitSpecify=off  UpperLimitBound=90  UpperLimitBoundUnits=deg  UpperLimitStiffness=1e4  UpperLimitStiffnessUnits=N*m/deg  UpperLimitDamping=10  UpperLimitDampingUnits=N*m/(deg/s)  UpperLimitTransitionRegionWidth=0.1  UpperLimitTransitionRegionWidthUnits=deg  PositionTargetSpecify=on  PositionTargetPriority=High  PositionTargetValue=50  PositionTargetValueUnits=deg  VelocityTargetSpecify=off  VelocityTargetPriority=High  VelocityTargetValue=0  VelocityTargetValueUnits=deg/s
  Cylinder Base [Lower Joint] : PMIOPort  Side=Left
  Mounting Assembly : PMIOPort  Port=2  Side=Left
  tag scope: BuA=global, BuV=global, UA=global, UV=global
  wires:
  PS-Simulink Converter Upper/1 -> [UA]
  Bucket Command Selector/1 -> Upper Arm Assembly/1(Pressure [Bucket Joint])
  Control  Commands [u]/1 -> Upper Command Selector/1, Bucket Command Selector/1
  Upper Command Selector/1 -> Hydraulic Actuator Lower - Upper Arm/1
  PS-Simulink Converter Upper1/1 -> [BuA]
  PS-Simulink Converter Upper2/1 -> [BuV]
  PS-Simulink Converter Upper3/1 -> [UV]
  connections:
  Hydraulic Actuator Lower - Upper Arm/RConn1 -- Upper Arm to Actuator Joint/LConn1
  Bucket/RConn2 -- Arm-Bucket Joint/RConn1
  Bucket/RConn1 -- Crank-Bucket Joint/RConn1
  Upper Arm Assembly/RConn2 -- Arm-Bucket Joint/LConn1
  Upper Arm to Actuator Joint/RConn1 -- Upper Arm Assembly/LConn1
  PS-Simulink Converter Upper/LConn1 -- Upper-Lower Arm Joint/RConn2
  Upper Arm Assembly/RConn1 -- Crank-Bucket Joint/LConn1
  Lower Arm to Cylinder Base/RConn1 -- Hydraulic Actuator Lower - Upper Arm/LConn1
  Upper-Lower Arm Joint/RConn1 -- Upper Arm Assembly/LConn2
  Lower Arm Assembly/RConn1 -- Lower Arm to Cylinder Base/LConn1
  Lower Arm Assembly/LConn2 -- Mounting Assembly/RConn1
  Lower Arm Assembly/RConn2 -- Upper-Lower Arm Joint/LConn1
  Cylinder Base [Lower Joint]/RConn1 -- Lower Arm Assembly/LConn1
  PS-Simulink Converter Upper1/LConn1 -- Arm-Bucket Joint/RConn2
  PS-Simulink Converter Upper2/LConn1 -- Arm-Bucket Joint/RConn3
  PS-Simulink Converter Upper3/LConn1 -- Upper-Lower Arm Joint/RConn3
